simulink model "sewermodel_malmo_conceptual"  (R2017a)
settings: Solver=ode45  StartTime=0.0  StopTime=18  RelTol=1e-3
undefined symbols (not defined in the file or in its folder): amp, freq, gwbias, gwtemp, inf_onoff, noise_onoff, noise_std, nreservoirs, phase
settings Model: Creator=ielsaagi  LastModifiedBy=ielsaagi
settings DataIOCC: OutputOption=SpecifiedOutputTimes  OutputTimes=[0:5/(24*60):18]

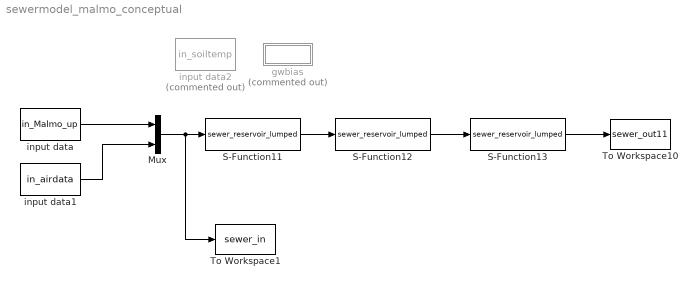
== system sewermodel_malmo_conceptual ==
  Mux : Mux  Inputs=2
  S-Function11 : S-Function  FunctionName=sewer_reservoir_lumped  Parameters=XINIT, PARAM_lumped, Qavg  SFunctionDeploymentMode=off  EnableBusSupport=off
  S-Function12 : S-Function  FunctionName=sewer_reservoir_lumped  Parameters=XINIT, PARAM_lumped, Qavg  SFunctionDeploymentMode=off  EnableBusSupport=off
  S-Function13 : S-Function  FunctionName=sewer_reservoir_lumped  Parameters=XINIT, PARAM_lumped, Qavg  SFunctionDeploymentMode=off  EnableBusSupport=off
  To Workspace1 : ToWorkspace  VariableName=sewer_in  SampleTime=-1
  To Workspace10 : ToWorkspace  VariableName=sewer_out11  SampleTime=-1
  gwbias : Subsystem  Commented=on
  input data : FromWorkspace  VariableName=in_Malmo_up  OutDataTypeStr=double  SampleTime=5/(24*60)  Interpolate=off  OutputAfterFinalValue=Cyclic repetition
  input data1 : FromWorkspace  VariableName=in_airdata  OutDataTypeStr=double  SampleTime=5/(24*60)  Interpolate=off  OutputAfterFinalValue=Cyclic repetition
  input data2 : FromWorkspace  Commented=on  VariableName=in_soiltemp  OutDataTypeStr=double  SampleTime=5/(24*60)  Interpolate=off  OutputAfterFinalValue=Cyclic repetition
  wires:
  input data/1 -> Mux/1
  input data1/1 -> Mux/2
  Mux/1 -> To Workspace1/1, S-Function11/1
  S-Function11/1 -> S-Function12/1
  S-Function12/1 -> S-Function13/1
  S-Function13/1 -> To Workspace10/1

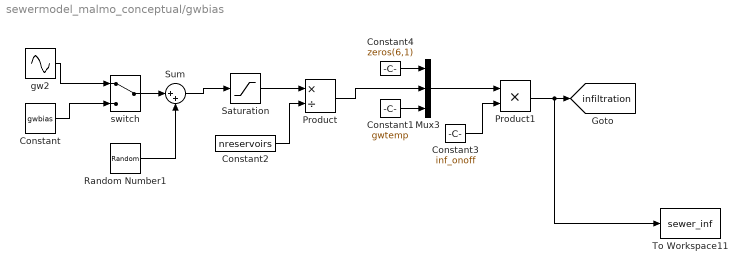
== system sewermodel_malmo_conceptual/gwbias ==
  Constant : Constant  Value=gwbias
  Constant1 : Constant  Value=gwtemp
  Constant2 : Constant  Value=nreservoirs
  Constant3 : Constant  Value=inf_onoff
  Constant4 : Constant  Value=zeros(6,1)
  Mux3 : Mux  Inputs=3
  Product : Product  Inputs=*/
  Product1 : Product
  Random Number1 : RandomNumber  Variance=noise_onoff*power(gwbias*noise_std,2)  Seed=44  SampleTime=1/96
  Saturation : Saturate  UpperLimit=gwbias*5  LowerLimit=0
  Sum : Sum  Inputs=|++
  To Workspace11 : ToWorkspace  VariableName=sewer_inf  SampleTime=1/96
  gw2 : Sin  Amplitude=gwbias*amp  Bias=gwbias  Frequency=freq  Phase=phase  SampleTime=0
  "switch " : ManualSwitch
  tag scope: infiltration=global
  wires:
  Random Number1/1 -> Sum/2
  gw2/1 -> "switch "/1
  Constant/1 -> "switch "/2
  "switch "/1 -> Sum/1
  Sum/1 -> Saturation/1
  Constant4/1 -> Mux3/1
  Saturation/1 -> Product/1
  Constant1/1 -> Mux3/3
  Constant2/1 -> Product/2
  Product/1 -> Mux3/2
  Mux3/1 -> Product1/1
  Constant3/1 -> Product1/2
  Product1/1 -> To Workspace11/1, [infiltration]
